simulink model "gaussian_filter"  (R2026a)
settings: Solver=VariableStepAuto
settings Model: Creator=svvb7  LastModifiedBy=svvb7

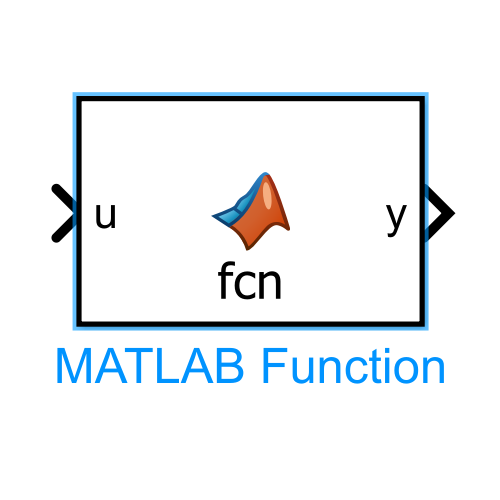
[thumbnail: Simulink's stored preview of the top-level diagram]
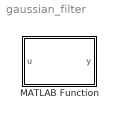
== system gaussian_filter ==
  MATLAB Function : MATLAB Function  TreatAsAtomicUnit=on

== matlab function gaussian_filter/MATLAB Function ==
  data: u input; y output
function y = fcn(u)
clc;
clear;
close all;

model = 'gaussian_filter';

new_system(model);

open_system(model);

% Input
add_block('simulink/Sources/In1', ...
    [model '/Pixel_Input']);

% Filter
add_block('simulink/Discrete/Discrete Filter', ...
    [model '/Gaussian_Block']);

% Output
add_block('simulink/Sinks/Out1', ...
    [model '/Filtered_Output']);

% Connect
add_line(model,'Pixel_Input/1','Gaussian_Block/1');

add_line(model,'Gaussian_Block/1','Filtered_Output/1');

save_system(model);

open_system(model);
